simulink model "RealAndSimulatedPlantBlock"  (R2021b)
settings: Solver=VariableStepAuto  StartTime=0.0  StopTime=10.0  RelTol=1e-3
values from neighbouring files (symbols this model uses):
  c = 0.2    [PlantParams.mat]    (also in params.m = 0.1)
  g = 9.81    [PlantParams.mat]    (also in params.m)
  J1 = 0.13138281053    [PlantParams.mat]    (also in params.m = 0.1314)
  Jz_bar = 0.0130765    [PlantParams.mat]    (also in params.m = 0.0131)
  lcg = 0.269778481013    [PlantParams.mat]    (also in params.m = 0.2698)
  m = 0.158    [PlantParams.mat]    (also in params.m)
  Rh = 0.37    [PlantParams.mat]
  rh = 0.37    [PlantParams.mat]    (also in params.m)
undefined symbols (not defined in the file or in its folder): gamma, l, theta_dot_init, theta_init
settings Model: Creator=samue  LastModifiedBy=samue

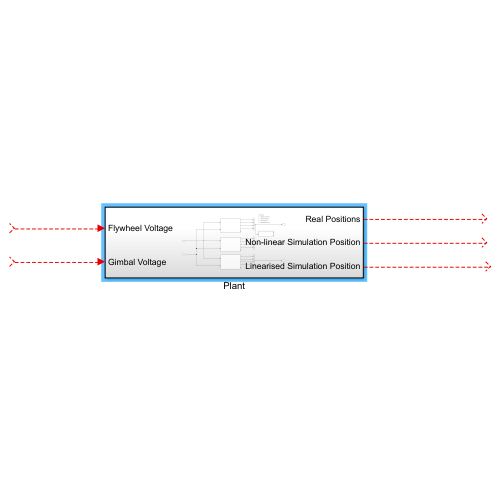
[thumbnail: Simulink's stored preview of the top-level diagram]
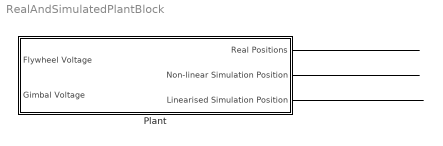
== system RealAndSimulatedPlantBlock ==
  Plant : Subsystem
  wires:
  ? -> Plant/1(Flywheel Voltage)
  ? -> Plant/2(Gimbal Voltage)
  Plant/1(Real Positions) -> ?
  Plant/2(Non-linear Simulation Position) -> ?
  Plant/3(Linearised Simulation Position) -> ?

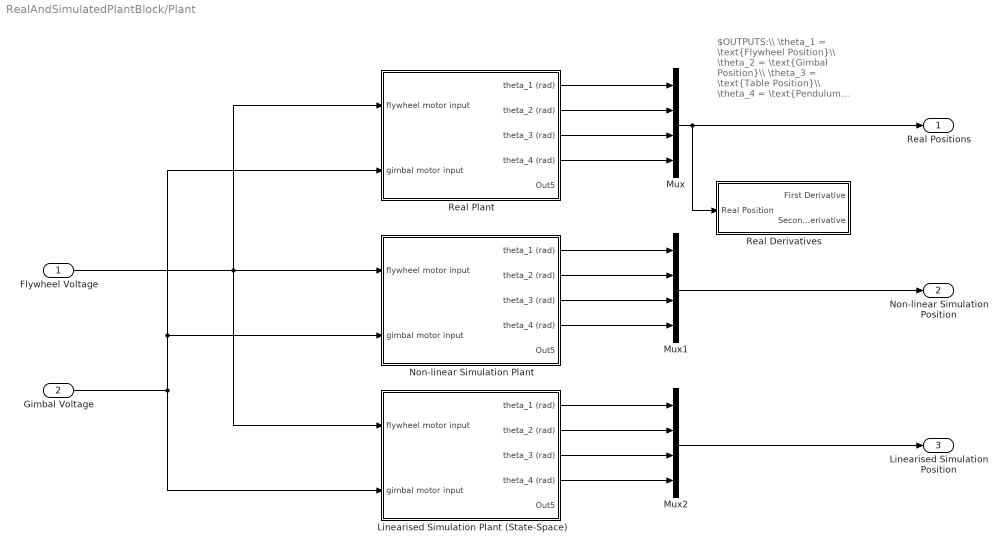
== system RealAndSimulatedPlantBlock/Plant ==
  note: $OUTPUTS:\\ \theta_1 = \text{Flywheel Position}\\ \theta_2 = \text{Gimbal Position}\\ \theta_3 = \text{Table Position}\\ \theta_4 = \text{Pendulum Position}\\$
  Flywheel Voltage : Inport
  Gimbal Voltage : Inport  Port=2
  Linearised Simulation Plant (State-Space) : Subsystem
  Mux : Mux
  Mux1 : Mux
  Mux2 : Mux
  Non-linear Simulation Plant : Subsystem
  Real Derivatives : Subsystem
  Real Plant : Subsystem
  Real Positions : Outport
  Non-linear Simulation Position : Outport  Port=2
  Linearised Simulation Position : Outport  Port=3
  wires:
  Linearised Simulation Plant (State-Space)/4(theta_4 (rad)) -> Mux2/4
  Non-linear Simulation Plant/1(theta_1 (rad)) -> Mux1/1
  Gimbal Voltage/1 -> Linearised Simulation Plant (State-Space)/2(gimbal motor input), Non-linear Simulation Plant/2(gimbal motor input), Real Plant/2(gimbal motor input)
  Non-linear Simulation Plant/2(theta_2 (rad)) -> Mux1/2
  Mux2/1 -> Linearised Simulation Position/1
  Linearised Simulation Plant (State-Space)/2(theta_2 (rad)) -> Mux2/2
  Flywheel Voltage/1 -> Linearised Simulation Plant (State-Space)/1(flywheel motor input), Non-linear Simulation Plant/1(flywheel motor input), Real Plant/1(flywheel motor input)
  Linearised Simulation Plant (State-Space)/3(theta_3 (rad)) -> Mux2/3
  Mux/1 -> Real Derivatives/1(Real Position), Real Positions/1
  Mux1/1 -> Non-linear Simulation Position/1
  Linearised Simulation Plant (State-Space)/1(theta_1 (rad)) -> Mux2/1
  Non-linear Simulation Plant/4(theta_4 (rad)) -> Mux1/4
  Real Plant/3(theta_3 (rad)) -> Mux/3
  Real Plant/1(theta_1 (rad)) -> Mux/1
  Real Plant/4(theta_4 (rad)) -> Mux/4
  Real Plant/2(theta_2 (rad)) -> Mux/2
  Non-linear Simulation Plant/3(theta_3 (rad)) -> Mux1/3

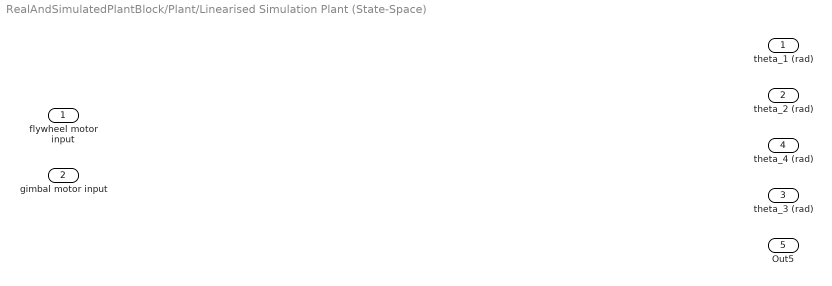
== system RealAndSimulatedPlantBlock/Plant/Linearised Simulation Plant (State-Space) ==
  flywheel motor input : Inport
  gimbal motor input : Inport  Port=2
  theta_1 (rad) : Outport
  theta_2 (rad) : Outport  Port=2
  theta_3 (rad) : Outport  Port=3
  theta_4 (rad) : Outport  Port=4
  Out5 : Outport  Port=5
  wires:
  ? -> theta_2 (rad)/1  "theta_2 (rad)"
  ? -> theta_1 (rad)/1  "theta_1 (rad)"
  ? -> theta_3 (rad)/1  "theta_3 (rad)"
  ? -> theta_4 (rad)/1  "theta_4 (rad)"

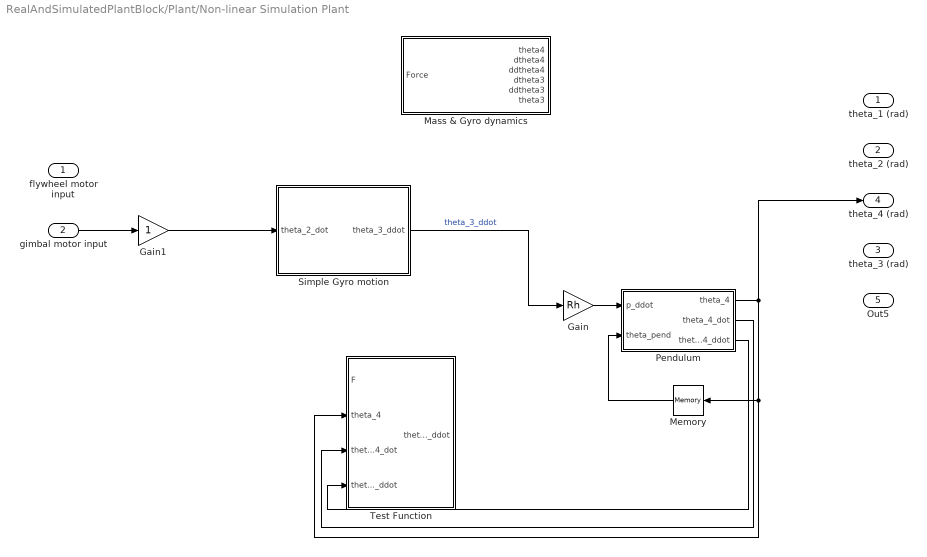
== system RealAndSimulatedPlantBlock/Plant/Non-linear Simulation Plant ==
  flywheel motor input : Inport
  gimbal motor input : Inport  Port=2
  Gain : Gain  Gain=Rh
  Gain1 : Gain
  Mass & Gyro dynamics : Subsystem
  Memory : Memory
  Pendulum : Subsystem
  Simple Gyro motion : MATLAB Function  TreatAsAtomicUnit=on
  Test Function : MATLAB Function  TreatAsAtomicUnit=on
  theta_1 (rad) : Outport
  theta_2 (rad) : Outport  Port=2
  theta_3 (rad) : Outport  Port=3
  theta_4 (rad) : Outport  Port=4
  Out5 : Outport  Port=5
  wires:
  ? -> theta_2 (rad)/1  "theta_2 (rad)"
  Gain/1 -> Pendulum/1(p_ddot)
  Simple Gyro motion/1(theta_3_ddot) -> Gain/1  "theta_3_ddot"
  Pendulum/3(theta_4_ddot) -> Test Function/4(theta_4_ddot)
  Pendulum/2(theta_4_dot) -> Test Function/3(theta_4_dot)
  Pendulum/1(theta_4) -> Test Function/2(theta_4), Memory/1, theta_4 (rad)/1
  Gain1/1 -> Simple Gyro motion/1(theta_2_dot)
  gimbal motor input/1 -> Gain1/1
  Memory/1 -> Pendulum/2(theta_pend)

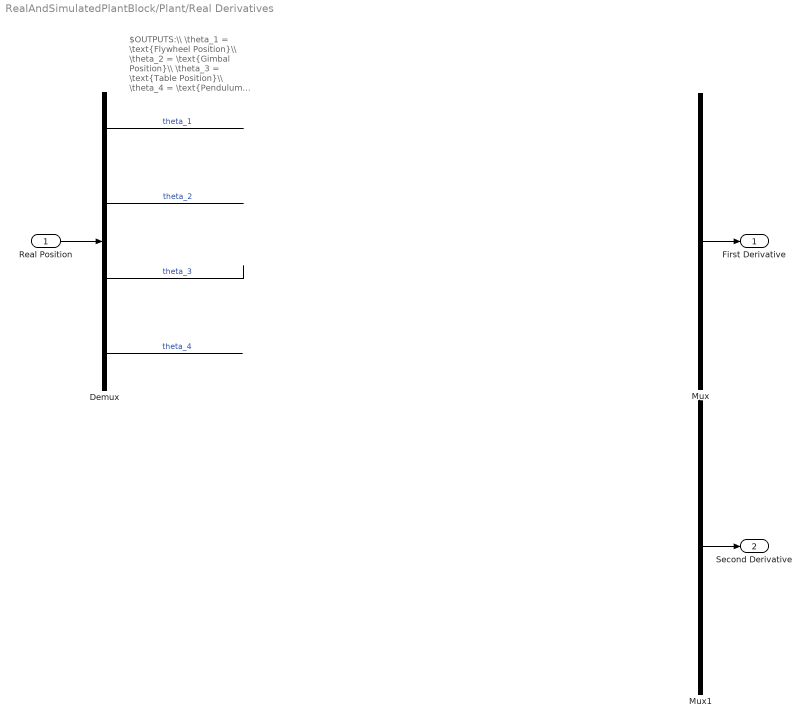
== system RealAndSimulatedPlantBlock/Plant/Real Derivatives ==
  note: $OUTPUTS:\\ \theta_1 = \text{Flywheel Position}\\ \theta_2 = \text{Gimbal Position}\\ \theta_3 = \text{Table Position}\\ \theta_4 = \text{Pendulum Position}\\$
  Real Position : Inport
  Demux : Demux
  Mux : Mux
  Mux1 : Mux
  First Derivative : Outport
  Second Derivative : Outport  Port=2
  wires:
  Real Position/1 -> Demux/1
  Demux/1 -> ?  "theta_1"
  Demux/2 -> ?  "theta_2"
  Demux/3 -> ?  "theta_3"
  Demux/4 -> ?  "theta_4"
  Mux/1 -> First Derivative/1
  Mux1/1 -> Second Derivative/1

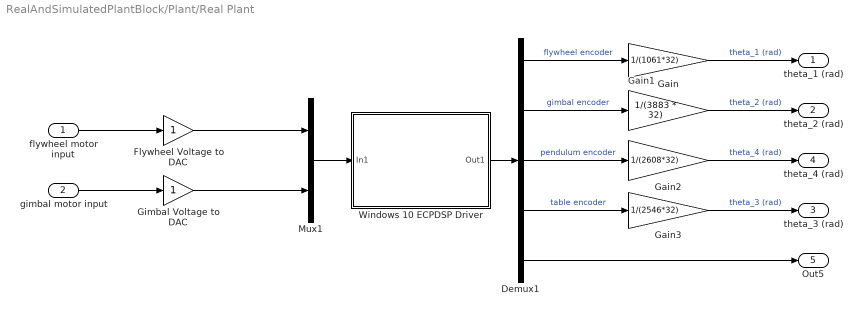
== system RealAndSimulatedPlantBlock/Plant/Real Plant ==
  flywheel motor input : Inport
  gimbal motor input : Inport  Port=2
  Demux1 : Demux  Outputs=5
      settings: DisplayOption=none
  Flywheel Voltage to DAC : Gain
  Gain : Gain  Gain=1/(1061*32)
  Gain1 : Gain  Gain=1/(3883 * 32)
  Gain2 : Gain  Gain=1/(2608*32)
  Gain3 : Gain  Gain=1/(2546*32)
  Gimbal Voltage to DAC : Gain
  Mux1 : Mux  Inputs=2
  Windows 10 ECPDSP Driver : Subsystem  mask{BaseAddr='0x3F00', STime=0.008, TimeOutPer=500, HWAccess=on}
      mask prompts: BaseAddr "Base I/O Address"; STime "Sample Time (Sec)"; TimeOutPer "Timeout Period (500 ~ 2000)"; HWAccess "Hardware Access"
      mask Display: color('black');disp('ECPDSP Driver\n upto\n 4 Encs(ADC Channels)\n and 2 Dacs')
  theta_1 (rad) : Outport
  theta_2 (rad) : Outport  Port=2
  theta_3 (rad) : Outport  Port=3
  theta_4 (rad) : Outport  Port=4
  Out5 : Outport  Port=5
  wires:
  Demux1/2 -> Gain1/1  "gimbal encoder"
  Demux1/1 -> Gain/1  "flywheel encoder"
  Demux1/3 -> Gain2/1  "pendulum encoder"
  Mux1/1 -> Windows 10 ECPDSP Driver/1(In1)
  Demux1/5 -> Out5/1
  Gain1/1 -> theta_2 (rad)/1  "theta_2 (rad)"
  gimbal motor input/1 -> Gimbal Voltage to DAC/1
  Demux1/4 -> Gain3/1  "table encoder"
  Windows 10 ECPDSP Driver/1(Out1) -> Demux1/1
  Gain/1 -> theta_1 (rad)/1  "theta_1 (rad)"
  flywheel motor input/1 -> Flywheel Voltage to DAC/1
  Gain3/1 -> theta_3 (rad)/1  "theta_3 (rad)"
  Gain2/1 -> theta_4 (rad)/1  "theta_4 (rad)"
  Flywheel Voltage to DAC/1 -> Mux1/1
  Gimbal Voltage to DAC/1 -> Mux1/2

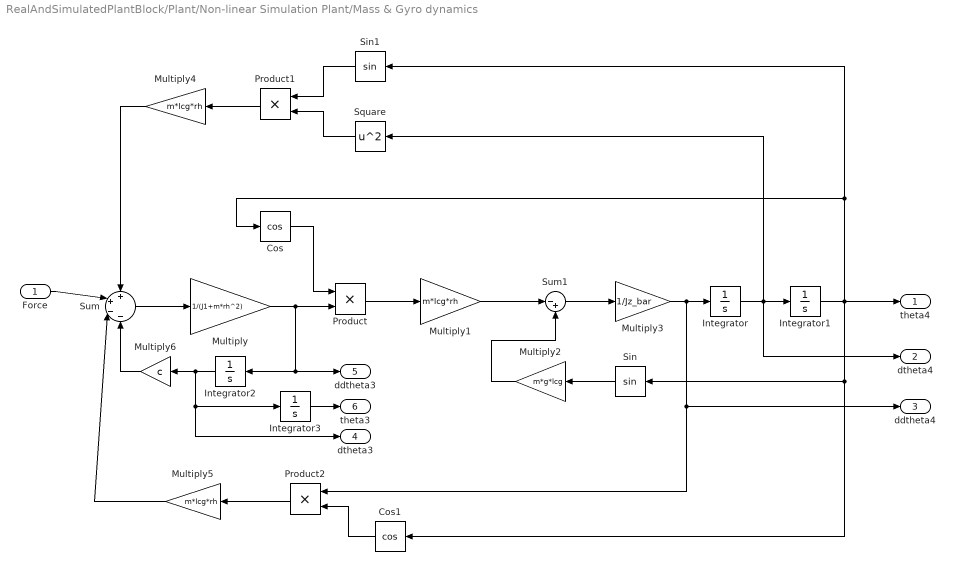
== system RealAndSimulatedPlantBlock/Plant/Non-linear Simulation Plant/Mass & Gyro dynamics ==
  Force : Inport
  Cos : Trigonometry  Operator=cos
  Cos1 : Trigonometry  Operator=cos
  Integrator : Integrator
  Integrator1 : Integrator  InitialCondition=pi
  Integrator2 : Integrator
  Integrator3 : Integrator
  Multiply : Gain  Gain=1/(J1+m*rh^2)
  Multiply1 : Gain  Gain=m*lcg*rh
  Multiply2 : Gain  Gain=m*g*lcg
  Multiply3 : Gain  Gain=1/Jz_bar
  Multiply4 : Gain  Gain=m*lcg*rh
  Multiply5 : Gain  Gain=m*lcg*rh
  Multiply6 : Gain  Gain=c
  Product : Product
  Product1 : Product
  Product2 : Product
  Sin : Trigonometry
  Sin1 : Trigonometry
  Square : Math  Operator=square  SaturateOnIntegerOverflow=on
  Sum : Sum  Inputs=++--
  Sum1 : Sum  Inputs=|-+
  theta4 : Outport
  dtheta4 : Outport  Port=2
  ddtheta4 : Outport  Port=3
  dtheta3 : Outport  Port=4
  ddtheta3 : Outport  Port=5
  theta3 : Outport  Port=6
  wires:
  Force/1 -> Sum/2
  Sum/1 -> Multiply/1
  Multiply/1 -> Integrator2/1, ddtheta3/1, Product/2
  Cos/1 -> Product/1
  Product/1 -> Multiply1/1
  Multiply1/1 -> Sum1/1
  Sin/1 -> Multiply2/1
  Multiply2/1 -> Sum1/2
  Sum1/1 -> Multiply3/1
  Multiply3/1 -> ddtheta4/1, Product2/1, Integrator/1
  Integrator/1 -> dtheta4/1, Square/1, Integrator1/1
  Integrator1/1 -> Cos1/1, Sin/1, theta4/1, Cos/1, Sin1/1
  Product1/1 -> Multiply4/1
  Multiply4/1 -> Sum/1
  Sin1/1 -> Product1/1
  Square/1 -> Product1/2
  Product2/1 -> Multiply5/1
  Multiply5/1 -> Sum/3
  Cos1/1 -> Product2/2
  Integrator2/1 -> Multiply6/1, dtheta3/1, Integrator3/1
  Multiply6/1 -> Sum/4
  Integrator3/1 -> theta3/1

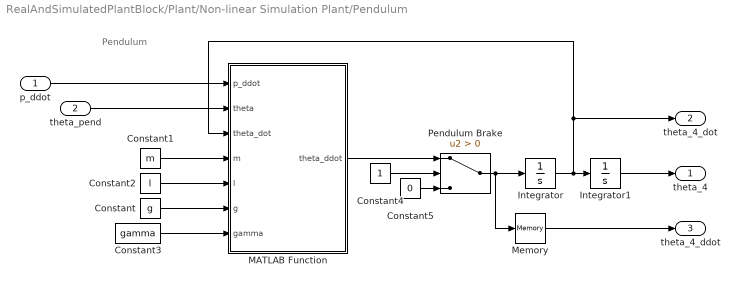
== system RealAndSimulatedPlantBlock/Plant/Non-linear Simulation Plant/Pendulum ==
  note: Pendulum
  p_ddot : Inport
  theta_pend : Inport  Port=2
  Constant : Constant  Value=g
  Constant1 : Constant  Value=m
  Constant2 : Constant  Value=l
  Constant3 : Constant  Value=gamma
  Constant4 : Constant
  Constant5 : Constant  Value=0
  Integrator : Integrator  InitialCondition=theta_dot_init
  Integrator1 : Integrator  InitialCondition=theta_init
  MATLAB Function : MATLAB Function  TreatAsAtomicUnit=on
  Memory : Memory
  Pendulum Brake : Switch  Criteria=u2 > Threshold
  theta_4 : Outport
  theta_4_dot : Outport  Port=2
  theta_4_ddot : Outport  Port=3
  wires:
  Integrator1/1 -> theta_4/1
  Pendulum Brake/1 -> Integrator/1, Memory/1
  Memory/1 -> theta_4_ddot/1
  theta_pend/1 -> MATLAB Function/2(theta)
  Integrator/1 -> MATLAB Function/3(theta_dot), theta_4_dot/1, Integrator1/1
  Constant1/1 -> MATLAB Function/4(m)
  Constant2/1 -> MATLAB Function/5(l)
  Constant/1 -> MATLAB Function/6(g)
  Constant3/1 -> MATLAB Function/7(gamma)
  p_ddot/1 -> MATLAB Function/1(p_ddot)
  MATLAB Function/1(theta_ddot) -> Pendulum Brake/1
  Constant4/1 -> Pendulum Brake/2
  Constant5/1 -> Pendulum Brake/3

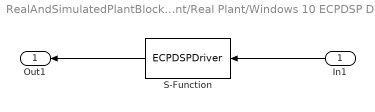
== system RealAndSimulatedPlantBlock/Plant/Real Plant/Windows 10 ECPDSP Driver ==
  In1 : Inport
  S-Function : S-Function  FunctionName=ECPDSPDriver  Parameters=BaseAddr,STime,TimeOutPer,HWAccess  SFunctionDeploymentMode=off  EnableBusSupport=off
  Out1 : Outport
  wires:
  In1/1 -> S-Function/1
  S-Function/1 -> Out1/1

== matlab function RealAndSimulatedPlantBlock/Plant/Non-linear Simulation Plant/Pendulum/MATLAB Function ==
  data: p_ddot input; theta_ddot output; theta input; theta_dot input; m input; l input; g input; gamma input
function theta_ddot = fcn(p_ddot, theta, theta_dot, m, l, g, gamma)

theta_ddot = (m*l*cos(theta)*p_ddot + m*g*l*sin(theta) - gamma*theta_dot)/(m*l^2);

== matlab function RealAndSimulatedPlantBlock/Plant/Non-linear Simulation Plant/Test Function ==
  data: F input; theta_3_ddot output; theta_4 input; theta_4_dot input; theta_4_ddot input
function theta_3_ddot = fcn(F, theta_4, theta_4_dot, theta_4_ddot)

theta_3_ddot = -(235565282109241125*theta_4_ddot - 6665327448508334080*F + 7532743254738029000*sin(theta_4))/(767863736466669568*cos(theta_4));

== matlab function RealAndSimulatedPlantBlock/Plant/Non-linear Simulation Plant/Simple Gyro motion ==
  data: theta_2_dot input; theta_3_ddot output
function theta_3_ddot = fcn(theta_2_dot)

theta_3_ddot = (40483834557657445*pi*theta_2_dot)/1817688811149124608;
